simulink model "StateObserverTest2"  (R2018b)
settings: Solver=VariableStepAuto  StartTime=0.0  StopTime=30  RelTol=1e-3
settings Model: Creator=mmbio  LastModifiedBy=mmbio

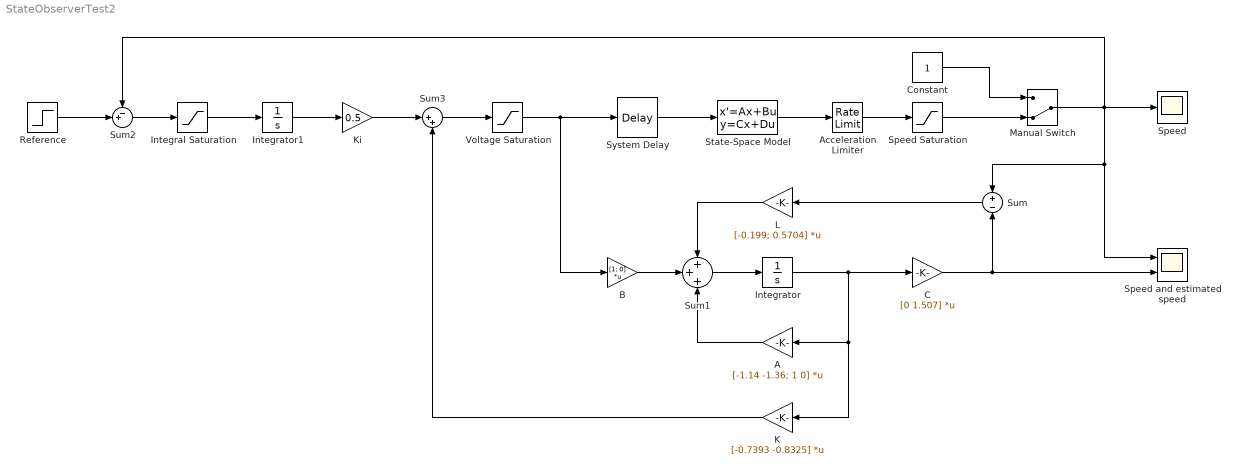
== system StateObserverTest2 ==
  A : Gain  Gain=[-1.14 -1.36; 1 0]  Multiplication=Matrix(K*u)
  Acceleration Limiter : RateLimiter  RisingSlewLimit=0.65  FallingSlewLimit=-0.65  SampleTimeMode=inherited
  B : Gain  Gain=[1; 0]  Multiplication=Matrix(K*u)
  C : Gain  Gain=[0 1.507]  Multiplication=Matrix(K*u)
  Constant : Constant
  Integral Saturation : Saturate  UpperLimit=5/0.5  LowerLimit=-5/0.5
  Integrator : Integrator
  Integrator1 : Integrator
  K : Gain  Gain=[-0.7393 -0.8325]  Multiplication=Matrix(K*u)
  Ki : Gain  Gain=0.5
  L : Gain  Gain=[-0.199; 0.5704]  Multiplication=Matrix(K*u)
  Manual Switch : ManualSwitch  CurrentSetting=0
  Reference : Step  SampleTime=0
  Speed : Scope
  Speed Saturation : Saturate  UpperLimit=1000  LowerLimit=0
  Speed and estimated speed : Scope  NumInputPorts=2
  State-Space Model : StateSpace  A=[-1.14 -1.36; 1 0]  B=[1; 0]  C=[0.0 1.507]  D=0  InitialCondition=0
  Sum : Sum  Inputs=+-
  Sum1 : Sum  Inputs=+++
  Sum2 : Sum  Inputs=-+|
  Sum3 : Sum  Inputs=|++
  System Delay : TransportDelay  DelayTime=0.45
  Voltage Saturation : Saturate  UpperLimit=5  LowerLimit=0
  wires:
  B/1 -> Sum1/2
  Voltage Saturation/1 -> System Delay/1, B/1
  K/1 -> Sum3/2
  Acceleration Limiter/1 -> Speed Saturation/1
  Reference/1 -> Sum2/2
  Sum2/1 -> Integral Saturation/1
  Manual Switch/1 -> Speed/1, Sum/1, Speed and estimated speed/1, Sum2/1
  System Delay/1 -> State-Space Model/1
  Ki/1 -> Sum3/1
  Sum3/1 -> Voltage Saturation/1
  Constant/1 -> Manual Switch/1
  Sum/1 -> L/1
  State-Space Model/1 -> Acceleration Limiter/1
  Sum1/1 -> Integrator/1
  C/1 -> Sum/2, Speed and estimated speed/2
  A/1 -> Sum1/3
  Integrator/1 -> K/1, A/1, C/1
  Integral Saturation/1 -> Integrator1/1
  L/1 -> Sum1/1
  Integrator1/1 -> Ki/1
  Speed Saturation/1 -> Manual Switch/2
